simulink model "base_simulink"  (R2021b)
settings: Solver=FixedStepAuto  StartTime=0.0  StopTime=6  FixedStep=0.00005  RelTol=1e-3
undefined symbols (not defined in the file): sigbuilder_block, twist, X, Y, Z
libraries: sm_lib x128, nesl_utility x42, slpidlib x16, ros2lib x8
(part 1 of 6)
settings Model: Creator=sanpo  LastModifiedBy=matas
settings DebuggingCC: AlgebraicLoopMsg=none

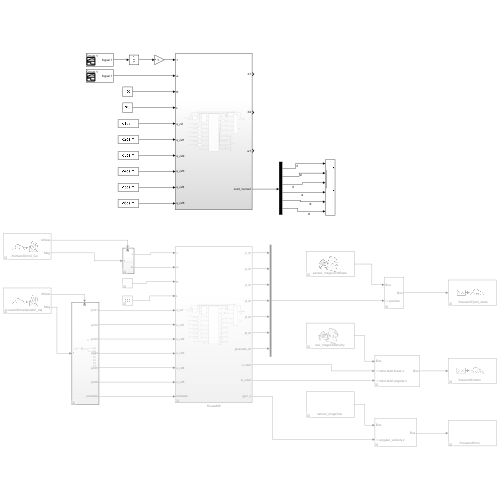
[thumbnail: Simulink's stored preview of the top-level diagram]
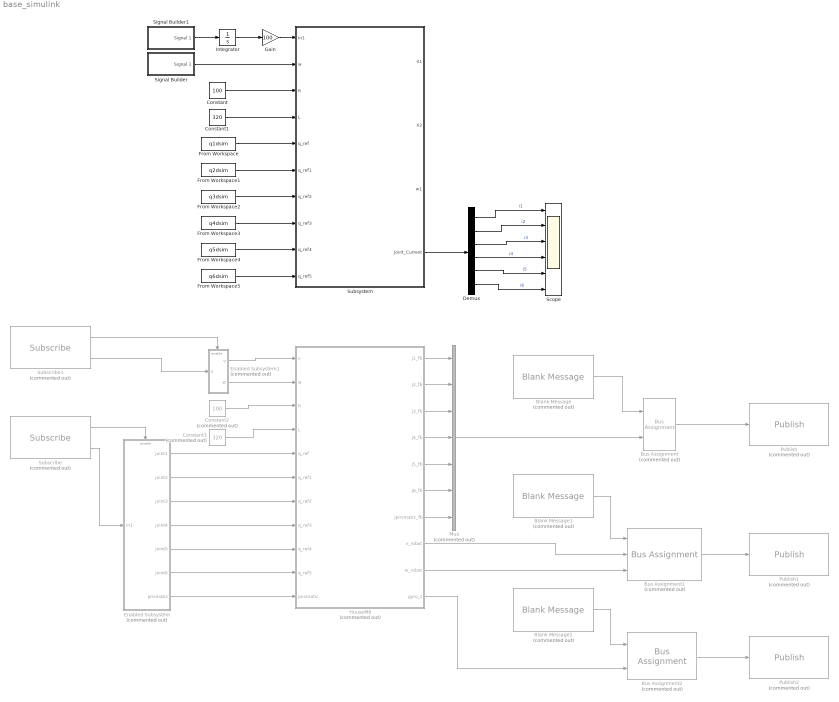
== system base_simulink ==
  Blank Message : ros2lib/Blank Message  Commented=on  messageClass=Message  entityType=sensor_msgs/JointState  messageType=sensor_msgs/JointState  SampleTime=0.01
      settings: SourceProductBaseCode=RR
  Blank Message1 : ros2lib/Blank Message  Commented=on  messageClass=Message  entityType=nav_msgs/Odometry  messageType=nav_msgs/Odometry  SampleTime=0.01
      settings: SourceProductBaseCode=RR
  Blank Message2 : ros2lib/Blank Message  Commented=on  messageClass=Message  entityType=sensor_msgs/Imu  messageType=geometry_msgs/Point  SampleTime=0.01
      settings: SourceProductBaseCode=RR
  Bus Assignment : BusAssignment  Commented=on  AssignedSignals=position
  Bus Assignment1 : BusAssignment  Commented=on  AssignedSignals=twist.twist.linear.x,twist.twist.angular.z
  Bus Assignment2 : BusAssignment  Commented=on  AssignedSignals=angular_velocity.z
  Constant : Constant  Value=100
  Constant1 : Constant  Value=320
  Constant2 : Constant  Commented=on  Value=100
  Constant3 : Constant  Commented=on  Value=320
  Demux : Demux  Outputs=6
  Enabled Subsystem : Subsystem  Commented=on
  Enabled Subsystem1 : Subsystem  Commented=on
  From Workspace : FromWorkspace  VariableName=q1dsim
  From Workspace1 : FromWorkspace  VariableName=q2dsim
  From Workspace2 : FromWorkspace  VariableName=q3dsim
  From Workspace3 : FromWorkspace  VariableName=q4dsim
  From Workspace4 : FromWorkspace  VariableName=q5dsim
  From Workspace5 : FromWorkspace  VariableName=q6dsim
  Gain : Gain  Gain=100
  HouseM8 : Subsystem  Commented=on
  Integrator : Integrator
  Mux : Mux  Commented=on  Inputs=7
  Publish : ros2lib/Publish  Commented=on  topicSource=Specify your own  topic=/housem8/joint_state  messageType=sensor_msgs/JointState  QOSHistory=Keep last  QOSDepth=1  QOSReliability=Reliable  QOSDurability=Volatile
      settings: SourceProductBaseCode=RR
  Publish1 : ros2lib/Publish  Commented=on  topicSource=Specify your own  topic=/housem8/odom  messageType=geometry_msgs/Point  QOSHistory=Keep last  QOSDepth=1  QOSReliability=Reliable  QOSDurability=Volatile
      settings: SourceProductBaseCode=RR
  Publish2 : ros2lib/Publish  Commented=on  topicSource=Specify your own  topic=/housem8/imu  messageType=geometry_msgs/Point  QOSHistory=Keep last  QOSDepth=1  QOSReliability=Reliable  QOSDurability=Volatile
      settings: SourceProductBaseCode=RR
  Scope : Scope  NumInputPorts=6
  Signal Builder : Subsystem  Tag=STV Subsys  LoadFcn=sigbuilder_block('load');  StartFcn=sigbuilder_block('start');  StopFcn=sigbuilder_block('stop');  ClipboardFcn=sigbuilder_block('clipboard');  mask(Sigbuilder block){tuvar=[0:10]}
      mask help: Simulink:masks:SigbuilderBlock_MD
      mask init:
      | if ~strcmp(get_param(bdroot(gcbh),'SimulationStatus'),'stopped') tuvar = sigbuilder_block('maskInit'); end
      settings: CopyFcn=sigbuilder_block('copy');  DeleteFcn=sigbuilder_block('delete');  ModelCloseFcn=sigbuilder_block('modelClose');  PreSaveFcn=sigbuilder_block('preSave');  PauseFcn=sigbuilder_block('pause');  ContinueFcn=sigbuilder_block('continue');  NameChangeFcn=sigbuilder_block('namechange');  OpenFcn=sigbuilder_block('open',[543 204.75 550.5 399.75 ]);  CloseFcn=sigbuilder_block('close');
      mask Display: plot(0, 0, 100, 100,[2, 2, 32, 32, 2], [68, 8, 8, 68, 68],[32, 2], [38, 38], [32, 19, 2],[53, 60, 44], [32, 17, 17, 2],[16, 16, 31, 31]);txt = getActiveGroup(gcbh);text(2, 100, txt,'verticalAlignment', 'top');
  Signal Builder1 : Subsystem  Tag=STV Subsys  LoadFcn=sigbuilder_block('load');  StartFcn=sigbuilder_block('start');  StopFcn=sigbuilder_block('stop');  ClipboardFcn=sigbuilder_block('clipboard');  mask(Sigbuilder block){tuvar=[0:10]}
      mask help: Simulink:masks:SigbuilderBlock_MD
      mask init:
      | if ~strcmp(get_param(bdroot(gcbh),'SimulationStatus'),'stopped') tuvar = sigbuilder_block('maskInit'); end
      settings: CopyFcn=sigbuilder_block('copy');  DeleteFcn=sigbuilder_block('delete');  ModelCloseFcn=sigbuilder_block('modelClose');  PreSaveFcn=sigbuilder_block('preSave');  PauseFcn=sigbuilder_block('pause');  ContinueFcn=sigbuilder_block('continue');  NameChangeFcn=sigbuilder_block('namechange');  OpenFcn=sigbuilder_block('open',[543 204.75 550.5 399.75 ]);  CloseFcn=sigbuilder_block('close');
      mask Display: plot(0, 0, 100, 100,[2, 2, 32, 32, 2], [68, 8, 8, 68, 68],[32, 2], [38, 38], [32, 19, 2],[53, 60, 44], [32, 17, 17, 2],[16, 16, 31, 31]);txt = getActiveGroup(gcbh);text(2, 100, txt,'verticalAlignment', 'top');
  Subscribe : ros2lib/Subscribe  Commented=on  topicSource=Specify your own  topic=/housem8/manipulator_traj  messageType=trajectory_msgs/MultiDOFJointTrajectory  sampleTime=0.01  QOSHistory=Keep last  QOSDepth=1  QOSReliability=Reliable  QOSDurability=Volatile
      settings: SourceProductBaseCode=RR
  Subscribe1 : ros2lib/Subscribe  Commented=on  topicSource=Specify your own  topic=/homem8/cmd_vel  messageType=geometry_msgs/Twist  sampleTime=0.01  QOSHistory=Keep last  QOSDepth=1  QOSReliability=Reliable  QOSDurability=Volatile
      settings: SourceProductBaseCode=RR
  Subsystem : Subsystem
  wires:
  Integrator/1 -> Gain/1
  Signal Builder1/1(Signal 1) -> Integrator/1
  Gain/1 -> Subsystem/1(In1)
  Signal Builder/1(Signal 1) -> Subsystem/2(w)
  Constant/1 -> Subsystem/3(R)
  Constant1/1 -> Subsystem/4(L)
  From Workspace/1 -> Subsystem/5(q_ref)
  From Workspace1/1 -> Subsystem/6(q_ref1)
  From Workspace2/1 -> Subsystem/7(q_ref2)
  From Workspace3/1 -> Subsystem/8(q_ref3)
  From Workspace4/1 -> Subsystem/9(q_ref4)
  From Workspace5/1 -> Subsystem/10(q_ref5)
  Subscribe/2 -> Enabled Subsystem/1(In1)
  Subscribe/1 -> Enabled Subsystem/Enable
  Constant3/1 -> HouseM8/4(L)
  Constant2/1 -> HouseM8/3(R)
  Enabled Subsystem/7(prismatic) -> HouseM8/11(prismatic)
  Enabled Subsystem/1(่่joint1) -> HouseM8/5(q_ref)
  Enabled Subsystem/2(joint2) -> HouseM8/6(q_ref1)
  Enabled Subsystem/3(joint3) -> HouseM8/7(q_ref2)
  Enabled Subsystem/4(joint4) -> HouseM8/8(q_ref3)
  Enabled Subsystem/5(joint5) -> HouseM8/9(q_ref4)
  Enabled Subsystem/6(joint6) -> HouseM8/10(q_ref5)
  Blank Message/1 -> Bus Assignment/1
  Bus Assignment/1 -> Publish/1
  Bus Assignment1/1 -> Publish1/1
  Blank Message1/1 -> Bus Assignment1/1
  Bus Assignment2/1 -> Publish2/1
  Blank Message2/1 -> Bus Assignment2/1
  HouseM8/10(gyro_z) -> Bus Assignment2/2
  HouseM8/1(j1_fb) -> Mux/1
  HouseM8/3(j3_fb) -> Mux/3
  HouseM8/2(j2_fb) -> Mux/2
  HouseM8/4(j4_fb) -> Mux/4
  HouseM8/5(j5_fb) -> Mux/5
  HouseM8/6(j6_fb) -> Mux/6
  HouseM8/7(jprismatic_fb) -> Mux/7
  Mux/1 -> Bus Assignment/2
  HouseM8/8(v_robot) -> Bus Assignment1/2
  HouseM8/9(w_robot) -> Bus Assignment1/3
  Subscribe1/1 -> Enabled Subsystem1/Enable
  Subscribe1/2 -> Enabled Subsystem1/1(In1)
  Enabled Subsystem1/1(v) -> HouseM8/1(v)
  Enabled Subsystem1/2(w) -> HouseM8/2(w)
  Subsystem/4(Joint_Current) -> Demux/1
  Demux/1 -> Scope/1  "i1"
  Demux/2 -> Scope/2  "i2"
  Demux/3 -> Scope/3  "i3"
  Demux/4 -> Scope/4  "i4"
  Demux/5 -> Scope/5  "i5"
  Demux/6 -> Scope/6  "i6"

== system base_simulink/Enabled Subsystem ==
  In1 : Inport
  Enable : EnablePort
  Bus Selector : BusSelector  DialogController=Simulink.DDGSource_BusSelector  OutputSignals=x,y
  ่่joint1 : Outport  VectorParamsAs1DForOutWhenUnconnected=off
  joint2 : Outport  Port=2  VectorParamsAs1DForOutWhenUnconnected=off
  joint3 : Outport  Port=3  VectorParamsAs1DForOutWhenUnconnected=off
  joint4 : Outport  Port=4  VectorParamsAs1DForOutWhenUnconnected=off
  joint5 : Outport  Port=5  VectorParamsAs1DForOutWhenUnconnected=off
  joint6 : Outport  Port=6  VectorParamsAs1DForOutWhenUnconnected=off
  prismatic : Outport  Port=7  VectorParamsAs1DForOutWhenUnconnected=off
  wires:
  In1/1 -> Bus Selector/1
  Bus Selector/1 -> ่่joint1/1  "<x>"
  Bus Selector/2 -> joint2/1  "<y>"

== system base_simulink/Enabled Subsystem1 ==
  In1 : Inport
  Enable : EnablePort
  Bus Selector : BusSelector  DialogController=Simulink.DDGSource_BusSelector  OutputSignals=x,y
  v : Outport  VectorParamsAs1DForOutWhenUnconnected=off
  w : Outport  Port=2  VectorParamsAs1DForOutWhenUnconnected=off
  wires:
  In1/1 -> Bus Selector/1
  Bus Selector/1 -> v/1  "<x>"
  Bus Selector/2 -> w/1  "<y>"

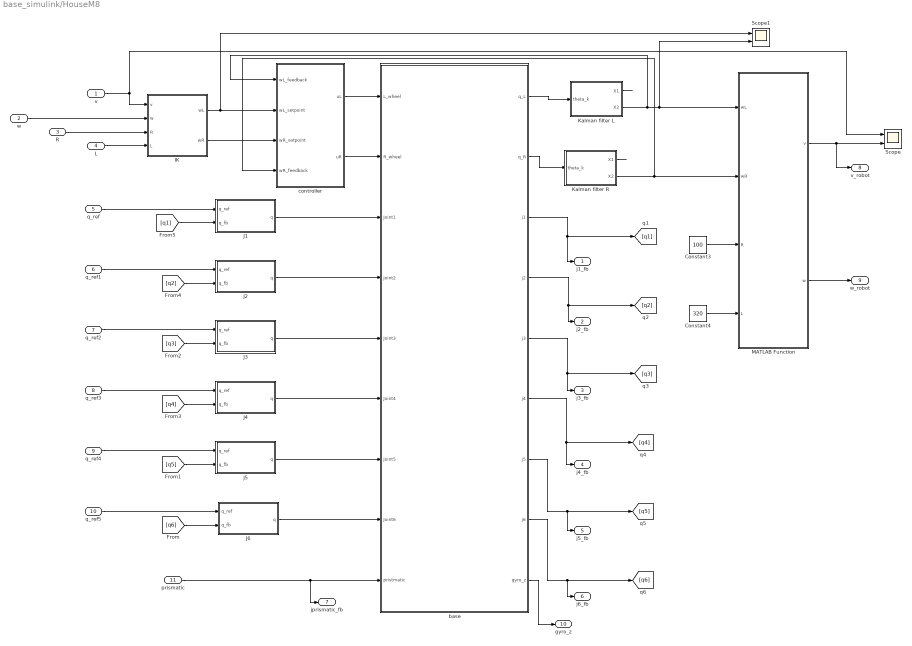
== system base_simulink/HouseM8 ==
  v : Inport
  w : Inport  Port=2
  R : Inport  Port=3
  L : Inport  Port=4
  q_ref : Inport  Port=5
  q_ref1 : Inport  Port=6
  q_ref2 : Inport  Port=7
  q_ref3 : Inport  Port=8
  q_ref4 : Inport  Port=9
  q_ref5 : Inport  Port=10
  prismatic : Inport  Port=11
  Constant3 : Constant  Value=100
  Constant4 : Constant  Value=320
  IK : MATLAB Function  TreatAsAtomicUnit=on
  J1 : Subsystem
  J2 : Subsystem
  J3 : Subsystem
  J4 : Subsystem
  J5 : Subsystem
  J6 : Subsystem
  Kalman filter L : Subsystem
  Kalman filter R : Subsystem
  MATLAB Function : MATLAB Function  TreatAsAtomicUnit=on
  Scope : Scope  NumInputPorts=2
  Scope1 : Scope  NumInputPorts=2
  base : Subsystem
  controller : Subsystem
  j1_fb : Outport
  j2_fb : Outport  Port=2
  j3_fb : Outport  Port=3
  j4_fb : Outport  Port=4
  j5_fb : Outport  Port=5
  j6_fb : Outport  Port=6
  jprismatic_fb : Outport  Port=7
  v_robot : Outport  Port=8
  w_robot : Outport  Port=9
  gyro_z : Outport  Port=10
  wires:
  base/4(j2) -> j2_fb/1, [q2]
  v/1 -> Scope/1, IK/1(v)
  IK/1(wL) -> Scope1/1, controller/2(wL_setpoint)
  Constant4/1 -> MATLAB Function/4(L)
  J6/1(q) -> base/8(Joint6)
  Kalman filter R/2(X2) -> controller/4(wR_feedback), MATLAB Function/2(wR)
  J1/1(q) -> base/3(Joint1)
  controller/2(uR) -> base/2(R_wheel)
  Kalman filter L/2(X2) -> Scope1/2, MATLAB Function/1(wL), controller/1(wL_feedback)
  base/8(j6) -> j6_fb/1, [q6]
  MATLAB Function/1(v) -> v_robot/1, Scope/2
  base/5(j3) -> j3_fb/1, [q3]
  q_ref2/1 -> J3/1(q_ref)
  base/2(q_R) -> Kalman filter R/1(theta_k)
  L/1 -> IK/4(L)
  J3/1(q) -> base/5(Joint3)
  Constant3/1 -> MATLAB Function/3(R)
  base/1(q_L) -> Kalman filter L/1(theta_k)
  q_ref/1 -> J1/1(q_ref)
  q_ref1/1 -> J2/1(q_ref)
  IK/2(wR) -> controller/3(wR_setpoint)
  Kalman filter L/1(X1) -> ?
  base/3(j1) -> j1_fb/1, [q1]
  prismatic/1 -> jprismatic_fb/1, base/9(pristmatic)
  [q1] -> J1/2(q_fb)
  q_ref5/1 -> J6/1(q_ref)
  base/6(j4) -> j4_fb/1, [q4]
  controller/1(uL) -> base/1(L_wheel)
  [q5] -> J5/2(q_fb)
  J4/1(q) -> base/6(Joint4)
  base/7(j5) -> j5_fb/1, [q5]
  [q2] -> J2/2(q_fb)
  [q3] -> J3/2(q_fb)
  J2/1(q) -> base/4(Joint2)
  Kalman filter R/1(X1) -> ?
  J5/1(q) -> base/7(Joint5)
  [q4] -> J4/2(q_fb)
  [q6] -> J6/2(q_fb)
  R/1 -> IK/3(R)
  w/1 -> IK/2(w)
  q_ref4/1 -> J5/1(q_ref)
  q_ref3/1 -> J4/1(q_ref)
  MATLAB Function/2(w) -> w_robot/1
  base/9(gyro_z) -> gyro_z/1

== system base_simulink/Signal Builder ==
  Demux : Demux  Tag=STV Demux  Outputs=1
      settings: DisplayOption=none
  FromWs : FromWorkspace  Tag=STV FromWs  VariableName=tuvar
      SigBuilderData=|
      | common.afterFinalStr = 'Extrapolate'
      | common.sampleTime = 0
      | dataSet.timeRange = [0 10]
      | dataSet.name = 'Group 1'
      | sbobj.Groups.Name = 'Group 1'
      | sbobj.Groups.Signals.Name = 'Signal 1'
      | sbobj.Groups.Signals.XData = [0 2 3 4 5 6 10]
      | sbobj.Groups.Signals.YData = [0 0 1 1 0 0 -1]
      | sbobj.Groups.TimeRange = [0 10]
  Signal 1 : Outport  Tag=STV Outport
  wires:
  Demux/1 -> Signal 1/1
  FromWs/1 -> Demux/1

== system base_simulink/Signal Builder1 ==
  Demux : Demux  Tag=STV Demux  Outputs=1
      settings: DisplayOption=none
  FromWs : FromWorkspace  Tag=STV FromWs  VariableName=tuvar
      SigBuilderData=|
      | common.afterFinalStr = 'Extrapolate'
      | common.sampleTime = 0
      | dataSet.timeRange = [0 10]
      | dataSet.name = 'Group 1'
      | sbobj.Groups.Name = 'Group 1'
      | sbobj.Groups.Signals.Name = 'Signal 1'
      | sbobj.Groups.Signals.XData = [0 0.5 6 10]
      | sbobj.Groups.Signals.YData = [5e-10 0.5 1 0]
  Signal 1 : Outport  Tag=STV Outport
  wires:
  FromWs/1 -> Demux/1
  Demux/1 -> Signal 1/1

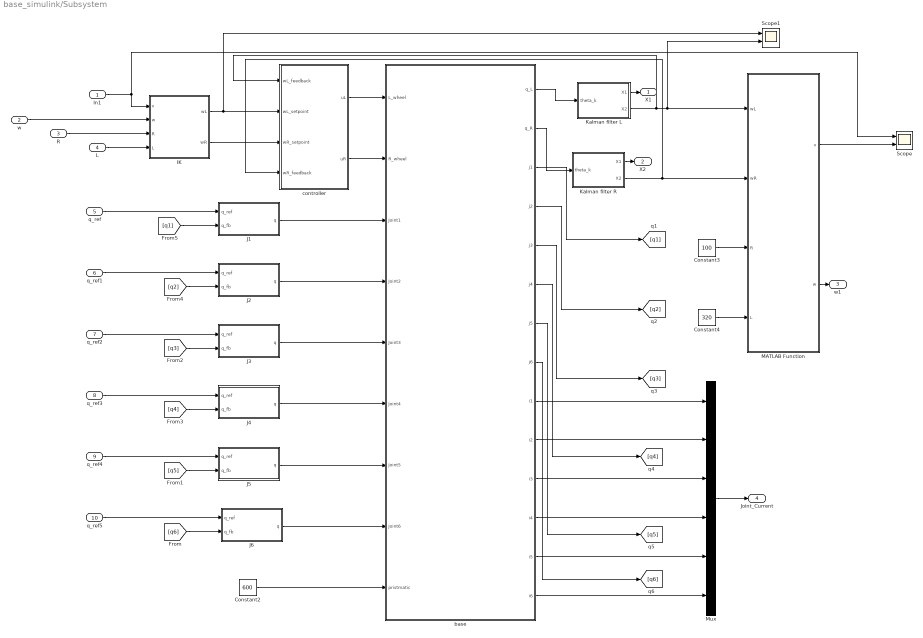
== system base_simulink/Subsystem ==
  In1 : Inport
  w : Inport  Port=2
  R : Inport  Port=3
  L : Inport  Port=4
  q_ref : Inport  Port=5
  q_ref1 : Inport  Port=6
  q_ref2 : Inport  Port=7
  q_ref3 : Inport  Port=8
  q_ref4 : Inport  Port=9
  q_ref5 : Inport  Port=10
  Constant2 : Constant  Value=600
  Constant3 : Constant  Value=100
  Constant4 : Constant  Value=320
  IK : MATLAB Function  TreatAsAtomicUnit=on
  J1 : Subsystem
  J2 : Subsystem
  J3 : Subsystem
  J4 : Subsystem
  J5 : Subsystem
  J6 : Subsystem
  Kalman filter L : Subsystem
  Kalman filter R : Subsystem
  MATLAB Function : MATLAB Function  TreatAsAtomicUnit=on
  Mux : Mux  Inputs=6
  Scope : Scope  NumInputPorts=2
  Scope1 : Scope  NumInputPorts=2
  base : Subsystem
  controller : Subsystem
  X1 : Outport
  X2 : Outport  Port=2
  w1 : Outport  Port=3
  Joint_Current : Outport  Port=4
  wires:
  base/4(j2) -> [q2]
  In1/1 -> Scope/1, IK/1(v)
  IK/1(wL) -> Scope1/1, controller/2(wL_setpoint)
  Constant4/1 -> MATLAB Function/4(L)
  J6/1(q) -> base/8(Joint6)
  Kalman filter R/2(X2) -> controller/4(wR_feedback), MATLAB Function/2(wR)
  J1/1(q) -> base/3(Joint1)
  controller/2(uR) -> base/2(R_wheel)
  Kalman filter L/2(X2) -> Scope1/2, MATLAB Function/1(wL), controller/1(wL_feedback)
  base/8(j6) -> [q6]
  MATLAB Function/1(v) -> Scope/2
  base/5(j3) -> [q3]
  q_ref2/1 -> J3/1(q_ref)
  base/2(q_R) -> Kalman filter R/1(theta_k)
  L/1 -> IK/4(L)
  J3/1(q) -> base/5(Joint3)
  Constant3/1 -> MATLAB Function/3(R)
  base/1(q_L) -> Kalman filter L/1(theta_k)
  q_ref/1 -> J1/1(q_ref)
  q_ref1/1 -> J2/1(q_ref)
  IK/2(wR) -> controller/3(wR_setpoint)
  Kalman filter L/1(X1) -> X1/1
  base/3(j1) -> [q1]
  Constant2/1 -> base/9(pristmatic)
  [q1] -> J1/2(q_fb)
  q_ref5/1 -> J6/1(q_ref)
  base/6(j4) -> [q4]
  controller/1(uL) -> base/1(L_wheel)
  [q5] -> J5/2(q_fb)
  J4/1(q) -> base/6(Joint4)
  base/7(j5) -> [q5]
  [q2] -> J2/2(q_fb)
  [q3] -> J3/2(q_fb)
  J2/1(q) -> base/4(Joint2)
  Kalman filter R/1(X1) -> X2/1
  J5/1(q) -> base/7(Joint5)
  [q4] -> J4/2(q_fb)
  [q6] -> J6/2(q_fb)
  R/1 -> IK/3(R)
  w/1 -> IK/2(w)
  q_ref4/1 -> J5/1(q_ref)
  q_ref3/1 -> J4/1(q_ref)
  MATLAB Function/2(w) -> w1/1
  base/9(i1) -> Mux/1
  base/10(i2) -> Mux/2
  base/11(i3) -> Mux/3
  base/12(i4) -> Mux/4
  base/13(i5) -> Mux/5
  base/14(i6) -> Mux/6
  Mux/1 -> Joint_Current/1

== system base_simulink/HouseM8/J1 ==
  q_ref : Inport
  q_fb : Inport  Port=2
  PID Controller : slpidlib/PID Controller  Controller=PID  Form=Parallel  TimeDomain=Discrete-time  UseExternalTs=off  SampleTime=0.001  IntegratorMethod=Forward Euler  FilterMethod=Forward Euler  ControllerParametersSource=internal  P=80  I=30  D=10  UseFilter=on  N=100  TunerSelectOption=Transfer Function Based (PID Tuner App)  InitialConditionSource=internal  InitialConditionForIntegrator=0  InitialConditionForFilter=0  DifferentiatorICPrevScaledInput=0  ExternalReset=none  TrackingMode=off  Kt=1  LimitOutput=off  SatLimitsSource=internal  UpperSaturationLimit=inf  LowerSaturationLimit=-inf  LinearizeAsGain=on  AntiWindupMode=none  Kb=1  POutMin=[]  POutMax=[]  IOutMin=[]  IOutMax=[]  DOutMin=[]  DOutMax=[]  NOutMin=[]  NOutMax=[]  SumOutMin=[]  SumOutMax=[]  SaturationOutMin=[]  SaturationOutMax=[]  PParamMin=[]  PParamMax=[]  IParamMin=[]  IParamMax=[]  DParamMin=[]  DParamMax=[]  NParamMin=[]  NParamMax=[]  KbParamMin=[]  KbParamMax=[]  KtParamMin=[]  KtParamMax=[]  KbOutMin=[]  KbOutMax=[]  KtOutMin=[]  KtOutMax=[]  IntegratorOutMin=[]  IntegratorOutMax=[]  FilterOutMin=[]  FilterOutMax=[]  SumI1OutMin=[]  SumI1OutMax=[]  SumI2OutMin=[]  SumI2OutMax=[]  SumI3OutMin=[]  SumI3OutMax=[]  SumI4OutMin=[]  SumI4OutMax=[]  SumDOutMin=[]  SumDOutMax=[]  DifferentiatorOutMin=[]  DifferentiatorOutMax=[]  FilterDiffOutCoefMin=[]  FilterDiffOutCoefMax=[]  ReciprocalOutMin=[]  ReciprocalOutMax=[]  SumDenOutMin=[]  SumDenOutMax=[]  SumNumOutMin=[]  SumNumOutMax=[]  DivideOutMin=[]  DivideOutMax=[]  UdiffTsProdOutMin=[]  UdiffTsProdOutMax=[]  NTsProdOutMin=[]  NTsProdOutMax=[]  UintegralTsProdOutMin=[]  UintegralTsProdOutMax=[]  UngainTsProdOutMin=[]  UngainTsProdOutMax=[]  IntegratorContinuousStateAttributes=''  IntegratorStateMustResolveToSignalObject=off  IntegratorRTWStateStorageClass=Auto  FilterContinuousStateAttributes=''  FilterStateMustResolveToSignalObject=off  FilterRTWStateStorageClass=Auto  ParallelPVariant=InternalParameters  IdealPVariant=Disabled  IVariant=InternalParameters  DVariant=InternalParameters  IntegratorVariant=Discrete  SatVariant=Disabled  AWVariant=Passthrough  PCopyVariant=Disabled  TRVariant=Disabled  FdbkBlocksVariant=Forward  IdealPFdbkVariant=Disabled  SatFdbkVariant=Disabled  DerivativeFilterVariant=ForwardEulerFilter  NVariant=InternalParameters  NCopyVariant=Disabled  FilterICVariant=InternalICsFilter  IntegratorICVariant=InternalICs  ExternalResetVariant=Disabled  TRSumVariant=Passthrough  SumFdbkVariant=Disabled  SumVariant=Sum_PID  TsampFilterVariant=InternalTs  TsampNgainVariant=Passthrough  TsampIntegralVariant=Passthrough  ExternalSaturationOutDataTypeStr=Inherit: Same as second input
  Sum : Sum  Inputs=|+-
  q : Outport
  wires:
  PID Controller/1 -> q/1
  Sum/1 -> PID Controller/1
  q_ref/1 -> Sum/1
  q_fb/1 -> Sum/2

== system base_simulink/HouseM8/J2 ==
  q_ref : Inport
  q_fb : Inport  Port=2
  PID Controller : slpidlib/PID Controller  Controller=PID  Form=Parallel  TimeDomain=Discrete-time  UseExternalTs=off  SampleTime=0.001  IntegratorMethod=Forward Euler  FilterMethod=Forward Euler  ControllerParametersSource=internal  P=90  I=30  D=12  UseFilter=on  N=100  TunerSelectOption=Transfer Function Based (PID Tuner App)  InitialConditionSource=internal  InitialConditionForIntegrator=0  InitialConditionForFilter=0  DifferentiatorICPrevScaledInput=0  ExternalReset=none  TrackingMode=off  Kt=1  LimitOutput=off  SatLimitsSource=internal  UpperSaturationLimit=inf  LowerSaturationLimit=-inf  LinearizeAsGain=on  AntiWindupMode=none  Kb=1  POutMin=[]  POutMax=[]  IOutMin=[]  IOutMax=[]  DOutMin=[]  DOutMax=[]  NOutMin=[]  NOutMax=[]  SumOutMin=[]  SumOutMax=[]  SaturationOutMin=[]  SaturationOutMax=[]  PParamMin=[]  PParamMax=[]  IParamMin=[]  IParamMax=[]  DParamMin=[]  DParamMax=[]  NParamMin=[]  NParamMax=[]  KbParamMin=[]  KbParamMax=[]  KtParamMin=[]  KtParamMax=[]  KbOutMin=[]  KbOutMax=[]  KtOutMin=[]  KtOutMax=[]  IntegratorOutMin=[]  IntegratorOutMax=[]  FilterOutMin=[]  FilterOutMax=[]  SumI1OutMin=[]  SumI1OutMax=[]  SumI2OutMin=[]  SumI2OutMax=[]  SumI3OutMin=[]  SumI3OutMax=[]  SumI4OutMin=[]  SumI4OutMax=[]  SumDOutMin=[]  SumDOutMax=[]  DifferentiatorOutMin=[]  DifferentiatorOutMax=[]  FilterDiffOutCoefMin=[]  FilterDiffOutCoefMax=[]  ReciprocalOutMin=[]  ReciprocalOutMax=[]  SumDenOutMin=[]  SumDenOutMax=[]  SumNumOutMin=[]  SumNumOutMax=[]  DivideOutMin=[]  DivideOutMax=[]  UdiffTsProdOutMin=[]  UdiffTsProdOutMax=[]  NTsProdOutMin=[]  NTsProdOutMax=[]  UintegralTsProdOutMin=[]  UintegralTsProdOutMax=[]  UngainTsProdOutMin=[]  UngainTsProdOutMax=[]  IntegratorContinuousStateAttributes=''  IntegratorStateMustResolveToSignalObject=off  IntegratorRTWStateStorageClass=Auto  FilterContinuousStateAttributes=''  FilterStateMustResolveToSignalObject=off  FilterRTWStateStorageClass=Auto  ParallelPVariant=InternalParameters  IdealPVariant=Disabled  IVariant=InternalParameters  DVariant=InternalParameters  IntegratorVariant=Discrete  SatVariant=Disabled  AWVariant=Passthrough  PCopyVariant=Disabled  TRVariant=Disabled  FdbkBlocksVariant=Forward  IdealPFdbkVariant=Disabled  SatFdbkVariant=Disabled  DerivativeFilterVariant=ForwardEulerFilter  NVariant=InternalParameters  NCopyVariant=Disabled  FilterICVariant=InternalICsFilter  IntegratorICVariant=InternalICs  ExternalResetVariant=Disabled  TRSumVariant=Passthrough  SumFdbkVariant=Disabled  SumVariant=Sum_PID  TsampFilterVariant=InternalTs  TsampNgainVariant=Passthrough  TsampIntegralVariant=Passthrough  ExternalSaturationOutDataTypeStr=Inherit: Same as second input
  Scope : Scope  NumInputPorts=2
  Sum : Sum  Inputs=|+-
  q : Outport
  wires:
  PID Controller/1 -> q/1
  Sum/1 -> PID Controller/1
  q_ref/1 -> Scope/1, Sum/1
  q_fb/1 -> Scope/2, Sum/2

== system base_simulink/HouseM8/J3 ==
  q_ref : Inport
  q_fb : Inport  Port=2
  PID Controller : slpidlib/PID Controller  Controller=PID  Form=Parallel  TimeDomain=Discrete-time  UseExternalTs=off  SampleTime=0.001  IntegratorMethod=Forward Euler  FilterMethod=Forward Euler  ControllerParametersSource=internal  P=80  I=25  D=12  UseFilter=on  N=100  TunerSelectOption=Transfer Function Based (PID Tuner App)  InitialConditionSource=internal  InitialConditionForIntegrator=0  InitialConditionForFilter=0  DifferentiatorICPrevScaledInput=0  ExternalReset=none  TrackingMode=off  Kt=1  LimitOutput=off  SatLimitsSource=internal  UpperSaturationLimit=inf  LowerSaturationLimit=-inf  LinearizeAsGain=on  AntiWindupMode=none  Kb=1  POutMin=[]  POutMax=[]  IOutMin=[]  IOutMax=[]  DOutMin=[]  DOutMax=[]  NOutMin=[]  NOutMax=[]  SumOutMin=[]  SumOutMax=[]  SaturationOutMin=[]  SaturationOutMax=[]  PParamMin=[]  PParamMax=[]  IParamMin=[]  IParamMax=[]  DParamMin=[]  DParamMax=[]  NParamMin=[]  NParamMax=[]  KbParamMin=[]  KbParamMax=[]  KtParamMin=[]  KtParamMax=[]  KbOutMin=[]  KbOutMax=[]  KtOutMin=[]  KtOutMax=[]  IntegratorOutMin=[]  IntegratorOutMax=[]  FilterOutMin=[]  FilterOutMax=[]  SumI1OutMin=[]  SumI1OutMax=[]  SumI2OutMin=[]  SumI2OutMax=[]  SumI3OutMin=[]  SumI3OutMax=[]  SumI4OutMin=[]  SumI4OutMax=[]  SumDOutMin=[]  SumDOutMax=[]  DifferentiatorOutMin=[]  DifferentiatorOutMax=[]  FilterDiffOutCoefMin=[]  FilterDiffOutCoefMax=[]  ReciprocalOutMin=[]  ReciprocalOutMax=[]  SumDenOutMin=[]  SumDenOutMax=[]  SumNumOutMin=[]  SumNumOutMax=[]  DivideOutMin=[]  DivideOutMax=[]  UdiffTsProdOutMin=[]  UdiffTsProdOutMax=[]  NTsProdOutMin=[]  NTsProdOutMax=[]  UintegralTsProdOutMin=[]  UintegralTsProdOutMax=[]  UngainTsProdOutMin=[]  UngainTsProdOutMax=[]  IntegratorContinuousStateAttributes=''  IntegratorStateMustResolveToSignalObject=off  IntegratorRTWStateStorageClass=Auto  FilterContinuousStateAttributes=''  FilterStateMustResolveToSignalObject=off  FilterRTWStateStorageClass=Auto  ParallelPVariant=InternalParameters  IdealPVariant=Disabled  IVariant=InternalParameters  DVariant=InternalParameters  IntegratorVariant=Discrete  SatVariant=Disabled  AWVariant=Passthrough  PCopyVariant=Disabled  TRVariant=Disabled  FdbkBlocksVariant=Forward  IdealPFdbkVariant=Disabled  SatFdbkVariant=Disabled  DerivativeFilterVariant=ForwardEulerFilter  NVariant=InternalParameters  NCopyVariant=Disabled  FilterICVariant=InternalICsFilter  IntegratorICVariant=InternalICs  ExternalResetVariant=Disabled  TRSumVariant=Passthrough  SumFdbkVariant=Disabled  SumVariant=Sum_PID  TsampFilterVariant=InternalTs  TsampNgainVariant=Passthrough  TsampIntegralVariant=Passthrough  ExternalSaturationOutDataTypeStr=Inherit: Same as second input
  Scope : Scope  NumInputPorts=2
  Sum : Sum  Inputs=|+-
  q : Outport
  wires:
  PID Controller/1 -> q/1
  Sum/1 -> PID Controller/1
  q_ref/1 -> Scope/1, Sum/1
  q_fb/1 -> Scope/2, Sum/2

== system base_simulink/HouseM8/J4 ==
  q_ref : Inport
  q_fb : Inport  Port=2
  PID Controller : slpidlib/PID Controller  Controller=PID  Form=Parallel  TimeDomain=Discrete-time  UseExternalTs=off  SampleTime=0.001  IntegratorMethod=Forward Euler  FilterMethod=Forward Euler  ControllerParametersSource=internal  P=80  I=20  D=8  UseFilter=on  N=100  TunerSelectOption=Transfer Function Based (PID Tuner App)  InitialConditionSource=internal  InitialConditionForIntegrator=0  InitialConditionForFilter=0  DifferentiatorICPrevScaledInput=0  ExternalReset=none  TrackingMode=off  Kt=1  LimitOutput=off  SatLimitsSource=internal  UpperSaturationLimit=inf  LowerSaturationLimit=-inf  LinearizeAsGain=on  AntiWindupMode=none  Kb=1  POutMin=[]  POutMax=[]  IOutMin=[]  IOutMax=[]  DOutMin=[]  DOutMax=[]  NOutMin=[]  NOutMax=[]  SumOutMin=[]  SumOutMax=[]  SaturationOutMin=[]  SaturationOutMax=[]  PParamMin=[]  PParamMax=[]  IParamMin=[]  IParamMax=[]  DParamMin=[]  DParamMax=[]  NParamMin=[]  NParamMax=[]  KbParamMin=[]  KbParamMax=[]  KtParamMin=[]  KtParamMax=[]  KbOutMin=[]  KbOutMax=[]  KtOutMin=[]  KtOutMax=[]  IntegratorOutMin=[]  IntegratorOutMax=[]  FilterOutMin=[]  FilterOutMax=[]  SumI1OutMin=[]  SumI1OutMax=[]  SumI2OutMin=[]  SumI2OutMax=[]  SumI3OutMin=[]  SumI3OutMax=[]  SumI4OutMin=[]  SumI4OutMax=[]  SumDOutMin=[]  SumDOutMax=[]  DifferentiatorOutMin=[]  DifferentiatorOutMax=[]  FilterDiffOutCoefMin=[]  FilterDiffOutCoefMax=[]  ReciprocalOutMin=[]  ReciprocalOutMax=[]  SumDenOutMin=[]  SumDenOutMax=[]  SumNumOutMin=[]  SumNumOutMax=[]  DivideOutMin=[]  DivideOutMax=[]  UdiffTsProdOutMin=[]  UdiffTsProdOutMax=[]  NTsProdOutMin=[]  NTsProdOutMax=[]  UintegralTsProdOutMin=[]  UintegralTsProdOutMax=[]  UngainTsProdOutMin=[]  UngainTsProdOutMax=[]  IntegratorContinuousStateAttributes=''  IntegratorStateMustResolveToSignalObject=off  IntegratorRTWStateStorageClass=Auto  FilterContinuousStateAttributes=''  FilterStateMustResolveToSignalObject=off  FilterRTWStateStorageClass=Auto  ParallelPVariant=InternalParameters  IdealPVariant=Disabled  IVariant=InternalParameters  DVariant=InternalParameters  IntegratorVariant=Discrete  SatVariant=Disabled  AWVariant=Passthrough  PCopyVariant=Disabled  TRVariant=Disabled  FdbkBlocksVariant=Forward  IdealPFdbkVariant=Disabled  SatFdbkVariant=Disabled  DerivativeFilterVariant=ForwardEulerFilter  NVariant=InternalParameters  NCopyVariant=Disabled  FilterICVariant=InternalICsFilter  IntegratorICVariant=InternalICs  ExternalResetVariant=Disabled  TRSumVariant=Passthrough  SumFdbkVariant=Disabled  SumVariant=Sum_PID  TsampFilterVariant=InternalTs  TsampNgainVariant=Passthrough  TsampIntegralVariant=Passthrough  ExternalSaturationOutDataTypeStr=Inherit: Same as second input
  Scope : Scope  NumInputPorts=2
  Sum : Sum  Inputs=|+-
  q : Outport
  wires:
  PID Controller/1 -> q/1
  Sum/1 -> PID Controller/1
  q_ref/1 -> Scope/1, Sum/1
  q_fb/1 -> Scope/2, Sum/2

== system base_simulink/HouseM8/J5 ==
  q_ref : Inport
  q_fb : Inport  Port=2
  PID Controller : slpidlib/PID Controller  Controller=PID  Form=Parallel  TimeDomain=Discrete-time  UseExternalTs=off  SampleTime=0.001  IntegratorMethod=Forward Euler  FilterMethod=Forward Euler  ControllerParametersSource=internal  P=85  I=25  D=10  UseFilter=on  N=100  TunerSelectOption=Transfer Function Based (PID Tuner App)  InitialConditionSource=internal  InitialConditionForIntegrator=0  InitialConditionForFilter=0  DifferentiatorICPrevScaledInput=0  ExternalReset=none  TrackingMode=off  Kt=1  LimitOutput=off  SatLimitsSource=internal  UpperSaturationLimit=inf  LowerSaturationLimit=-inf  LinearizeAsGain=on  AntiWindupMode=none  Kb=1  POutMin=[]  POutMax=[]  IOutMin=[]  IOutMax=[]  DOutMin=[]  DOutMax=[]  NOutMin=[]  NOutMax=[]  SumOutMin=[]  SumOutMax=[]  SaturationOutMin=[]  SaturationOutMax=[]  PParamMin=[]  PParamMax=[]  IParamMin=[]  IParamMax=[]  DParamMin=[]  DParamMax=[]  NParamMin=[]  NParamMax=[]  KbParamMin=[]  KbParamMax=[]  KtParamMin=[]  KtParamMax=[]  KbOutMin=[]  KbOutMax=[]  KtOutMin=[]  KtOutMax=[]  IntegratorOutMin=[]  IntegratorOutMax=[]  FilterOutMin=[]  FilterOutMax=[]  SumI1OutMin=[]  SumI1OutMax=[]  SumI2OutMin=[]  SumI2OutMax=[]  SumI3OutMin=[]  SumI3OutMax=[]  SumI4OutMin=[]  SumI4OutMax=[]  SumDOutMin=[]  SumDOutMax=[]  DifferentiatorOutMin=[]  DifferentiatorOutMax=[]  FilterDiffOutCoefMin=[]  FilterDiffOutCoefMax=[]  ReciprocalOutMin=[]  ReciprocalOutMax=[]  SumDenOutMin=[]  SumDenOutMax=[]  SumNumOutMin=[]  SumNumOutMax=[]  DivideOutMin=[]  DivideOutMax=[]  UdiffTsProdOutMin=[]  UdiffTsProdOutMax=[]  NTsProdOutMin=[]  NTsProdOutMax=[]  UintegralTsProdOutMin=[]  UintegralTsProdOutMax=[]  UngainTsProdOutMin=[]  UngainTsProdOutMax=[]  IntegratorContinuousStateAttributes=''  IntegratorStateMustResolveToSignalObject=off  IntegratorRTWStateStorageClass=Auto  FilterContinuousStateAttributes=''  FilterStateMustResolveToSignalObject=off  FilterRTWStateStorageClass=Auto  ParallelPVariant=InternalParameters  IdealPVariant=Disabled  IVariant=InternalParameters  DVariant=InternalParameters  IntegratorVariant=Discrete  SatVariant=Disabled  AWVariant=Passthrough  PCopyVariant=Disabled  TRVariant=Disabled  FdbkBlocksVariant=Forward  IdealPFdbkVariant=Disabled  SatFdbkVariant=Disabled  DerivativeFilterVariant=ForwardEulerFilter  NVariant=InternalParameters  NCopyVariant=Disabled  FilterICVariant=InternalICsFilter  IntegratorICVariant=InternalICs  ExternalResetVariant=Disabled  TRSumVariant=Passthrough  SumFdbkVariant=Disabled  SumVariant=Sum_PID  TsampFilterVariant=InternalTs  TsampNgainVariant=Passthrough  TsampIntegralVariant=Passthrough  ExternalSaturationOutDataTypeStr=Inherit: Same as second input
  Scope : Scope  NumInputPorts=2
  Sum : Sum  Inputs=|+-
  q : Outport
  wires:
  PID Controller/1 -> q/1
  Sum/1 -> PID Controller/1
  q_ref/1 -> Scope/1, Sum/1
  q_fb/1 -> Scope/2, Sum/2

== system base_simulink/HouseM8/J6 ==
  q_ref : Inport
  q_fb : Inport  Port=2
  PID Controller : slpidlib/PID Controller  Controller=PID  Form=Parallel  TimeDomain=Discrete-time  UseExternalTs=off  SampleTime=0.001  IntegratorMethod=Forward Euler  FilterMethod=Forward Euler  ControllerParametersSource=internal  P=65  I=32  D=10  UseFilter=on  N=100  TunerSelectOption=Transfer Function Based (PID Tuner App)  InitialConditionSource=internal  InitialConditionForIntegrator=0  InitialConditionForFilter=0  DifferentiatorICPrevScaledInput=0  ExternalReset=none  TrackingMode=off  Kt=1  LimitOutput=off  SatLimitsSource=internal  UpperSaturationLimit=inf  LowerSaturationLimit=-inf  LinearizeAsGain=on  AntiWindupMode=none  Kb=1  POutMin=[]  POutMax=[]  IOutMin=[]  IOutMax=[]  DOutMin=[]  DOutMax=[]  NOutMin=[]  NOutMax=[]  SumOutMin=[]  SumOutMax=[]  SaturationOutMin=[]  SaturationOutMax=[]  PParamMin=[]  PParamMax=[]  IParamMin=[]  IParamMax=[]  DParamMin=[]  DParamMax=[]  NParamMin=[]  NParamMax=[]  KbParamMin=[]  KbParamMax=[]  KtParamMin=[]  KtParamMax=[]  KbOutMin=[]  KbOutMax=[]  KtOutMin=[]  KtOutMax=[]  IntegratorOutMin=[]  IntegratorOutMax=[]  FilterOutMin=[]  FilterOutMax=[]  SumI1OutMin=[]  SumI1OutMax=[]  SumI2OutMin=[]  SumI2OutMax=[]  SumI3OutMin=[]  SumI3OutMax=[]  SumI4OutMin=[]  SumI4OutMax=[]  SumDOutMin=[]  SumDOutMax=[]  DifferentiatorOutMin=[]  DifferentiatorOutMax=[]  FilterDiffOutCoefMin=[]  FilterDiffOutCoefMax=[]  ReciprocalOutMin=[]  ReciprocalOutMax=[]  SumDenOutMin=[]  SumDenOutMax=[]  SumNumOutMin=[]  SumNumOutMax=[]  DivideOutMin=[]  DivideOutMax=[]  UdiffTsProdOutMin=[]  UdiffTsProdOutMax=[]  NTsProdOutMin=[]  NTsProdOutMax=[]  UintegralTsProdOutMin=[]  UintegralTsProdOutMax=[]  UngainTsProdOutMin=[]  UngainTsProdOutMax=[]  IntegratorContinuousStateAttributes=''  IntegratorStateMustResolveToSignalObject=off  IntegratorRTWStateStorageClass=Auto  FilterContinuousStateAttributes=''  FilterStateMustResolveToSignalObject=off  FilterRTWStateStorageClass=Auto  ParallelPVariant=InternalParameters  IdealPVariant=Disabled  IVariant=InternalParameters  DVariant=InternalParameters  IntegratorVariant=Discrete  SatVariant=Disabled  AWVariant=Passthrough  PCopyVariant=Disabled  TRVariant=Disabled  FdbkBlocksVariant=Forward  IdealPFdbkVariant=Disabled  SatFdbkVariant=Disabled  DerivativeFilterVariant=ForwardEulerFilter  NVariant=InternalParameters  NCopyVariant=Disabled  FilterICVariant=InternalICsFilter  IntegratorICVariant=InternalICs  ExternalResetVariant=Disabled  TRSumVariant=Passthrough  SumFdbkVariant=Disabled  SumVariant=Sum_PID  TsampFilterVariant=InternalTs  TsampNgainVariant=Passthrough  TsampIntegralVariant=Passthrough  ExternalSaturationOutDataTypeStr=Inherit: Same as second input
  Scope : Scope  NumInputPorts=2
  Sum : Sum  Inputs=|+-
  q : Outport
  wires:
  PID Controller/1 -> q/1
  Sum/1 -> PID Controller/1
  q_ref/1 -> Scope/1, Sum/1
  q_fb/1 -> Scope/2, Sum/2

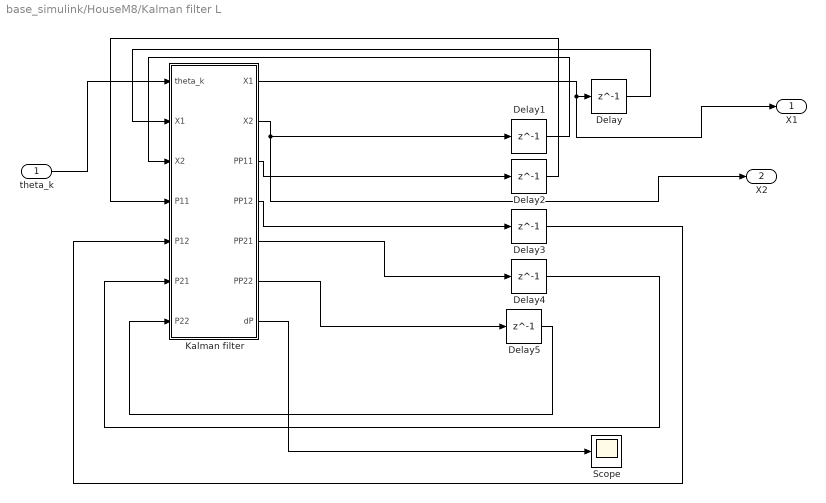
== system base_simulink/HouseM8/Kalman filter L ==
  theta_k : Inport
  Delay{,1..5} (6 alike) : Delay  DelayLength=1  SampleTime=0.0001
  Kalman filter : MATLAB Function  TreatAsAtomicUnit=on
  Scope : Scope
  X1 : Outport
  X2 : Outport  Port=2
  wires:
  Delay3/1 -> Kalman filter/5(P12)
  Kalman filter/3(PP11) -> Delay2/1
  Kalman filter/4(PP12) -> Delay3/1
  Delay2/1 -> Kalman filter/4(P11)
  Delay5/1 -> Kalman filter/7(P22)
  Delay/1 -> Kalman filter/2("X1 ")
  Kalman filter/1(X1) -> X1/1, Delay/1
  Kalman filter/5(PP21) -> Delay4/1
  Delay1/1 -> Kalman filter/3("X2 ")
  Delay4/1 -> Kalman filter/6(P21)
  theta_k/1 -> Kalman filter/1(theta_k)
  Kalman filter/2(X2) -> Delay1/1, X2/1
  Kalman filter/6(PP22) -> Delay5/1
  Kalman filter/7(dP) -> Scope/1

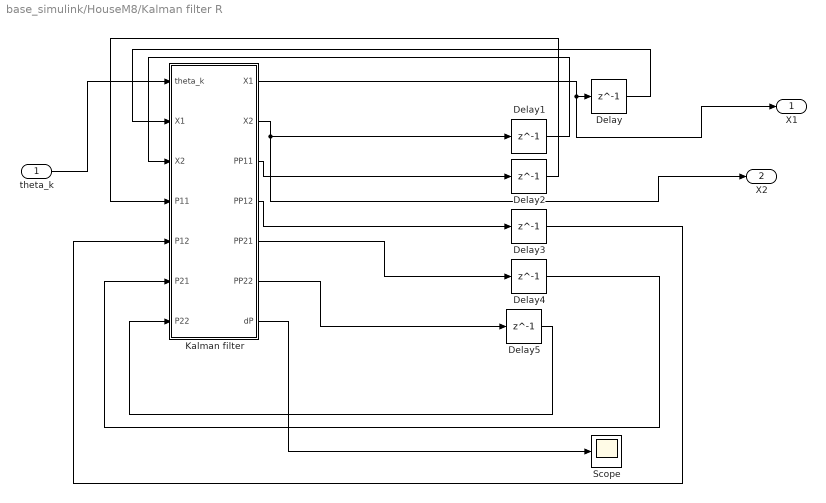
== system base_simulink/HouseM8/Kalman filter R ==
  theta_k : Inport
  Delay{,1..5} (6 alike) : Delay  DelayLength=1  SampleTime=0.0001
  Kalman filter : MATLAB Function  TreatAsAtomicUnit=on
  Scope : Scope
  X1 : Outport
  X2 : Outport  Port=2
  wires:
  Kalman filter/7(dP) -> Scope/1
  Kalman filter/6(PP22) -> Delay5/1
  Kalman filter/2(X2) -> X2/1, Delay1/1
  theta_k/1 -> Kalman filter/1(theta_k)
  Delay4/1 -> Kalman filter/6(P21)
  Delay1/1 -> Kalman filter/3("X2 ")
  Kalman filter/5(PP21) -> Delay4/1
  Kalman filter/1(X1) -> Delay/1, X1/1
  Delay/1 -> Kalman filter/2("X1 ")
  Delay5/1 -> Kalman filter/7(P22)
  Delay2/1 -> Kalman filter/4(P11)
  Kalman filter/4(PP12) -> Delay3/1
  Kalman filter/3(PP11) -> Delay2/1
  Delay3/1 -> Kalman filter/5(P12)

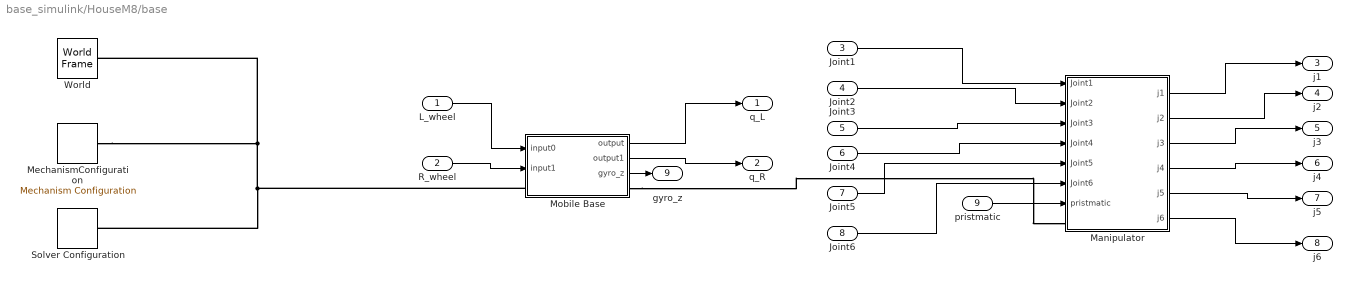
== system base_simulink/HouseM8/base ==
  L_wheel : Inport
  R_wheel : Inport  Port=2
  Joint1 : Inport  Port=3
  Joint2 : Inport  Port=4
  Joint3 : Inport  Port=5
  Joint4 : Inport  Port=6
  Joint5 : Inport  Port=7
  Joint6 : Inport  Port=8
  pristmatic : Inport  Port=9
  Manipulator : Subsystem
  MechanismConfiguration : sm_lib/Utilities/Mechanism Configuration  UniformGravity=Constant  GravityVector=[0 0 -9.80665]  GravityUnits=m/s^2  LinearizationDelta=0.001  JointModeTransitionNonlinearIterations=2
  Mobile Base : Subsystem
  Solver Configuration : nesl_utility/Solver Configuration  PhysicalDomain=network_engine_domain  SubClassName=solver  LeftPortType=input  RightPortType=generic  Tones=[]  Harmonics=[]  SimulateNoise=off  Profile=off  UseLocalSampling=off  EnableSwitchedLinearOptims=on  FrequencyDomain=off  UseCCode=off  RelTol=0.001  AbsTol=1e-06  MinStep=1e-09  ToWorkspace=off  RevertToSquareIcSolve=off  NumHomotopyIterations=100  PhasorMode=off  PhasorModeNumHarmonics=1  DoDC=off  ResidualTolerance=1e-09  UseLocalSolver=off  LocalSolverChoice=NE_BACKWARD_EULER_ADVANCER  LocalSolverSampleTime=0.001  DoFixedCost=off  MaxNonlinIter=3  MaxModeIter=2  ComputeImpulses=off  ImpulseIterations=2  LinearAlgebra=auto  EquationFormulation=NE_TIME_EF  DelaysMemoryBudget=1024  AutomaticFiltering=on  FilteringTimeConstant=0.001  PartitionStorageMethod=AS_NEEDED  PartitionMemoryBudget=1024  PartitionMethod=ROBUST
      settings: SourceProductBaseCode=PW,SS
  World : sm_lib/Frames and Transforms/World Frame
  q_L : Outport
  q_R : Outport  Port=2
  j1 : Outport  Port=3
  j2 : Outport  Port=4
  j3 : Outport  Port=5
  j4 : Outport  Port=6
  j5 : Outport  Port=7
  j6 : Outport  Port=8
  gyro_z : Outport  Port=9
  wires:
  L_wheel/1 -> Mobile Base/1(input0)
  R_wheel/1 -> Mobile Base/2(input1)
  Mobile Base/1(output) -> q_L/1
  Mobile Base/2(output1) -> q_R/1
  Joint1/1 -> Manipulator/1(Joint1)
  Joint2/1 -> Manipulator/2(Joint2)
  Joint3/1 -> Manipulator/3(Joint3)
  Joint4/1 -> Manipulator/4(Joint4)
  Joint5/1 -> Manipulator/5(Joint5)
  Joint6/1 -> Manipulator/6(Joint6)
  pristmatic/1 -> Manipulator/7(pristmatic)
  Manipulator/1(j1) -> j1/1
  Manipulator/2(j2) -> j2/1
  Manipulator/3(j3) -> j3/1
  Manipulator/4(j4) -> j4/1
  Manipulator/5(j5) -> j5/1
  Manipulator/6(j6) -> j6/1
  Mobile Base/3(gyro_z) -> gyro_z/1
  connections:
  Mobile Base/LConn1 -- Solver Configuration/RConn1 -- MechanismConfiguration/RConn1 -- World/RConn1
  Mobile Base/RConn1 -- Manipulator/LConn1

== system base_simulink/HouseM8/controller ==
  wL_feedback : Inport
  wL_setpoint : Inport  Port=2
  wR_setpoint : Inport  Port=3
  wR_feedback : Inport  Port=4
  PID Controller : slpidlib/PID Controller  Controller=PID  Form=Parallel  TimeDomain=Discrete-time  UseExternalTs=off  SampleTime=0.001  IntegratorMethod=Forward Euler  FilterMethod=Forward Euler  ControllerParametersSource=internal  P=1.5  I=0.6  D=1  UseFilter=on  N=100  TunerSelectOption=Transfer Function Based (PID Tuner App)  InitialConditionSource=internal  InitialConditionForIntegrator=0  InitialConditionForFilter=0  DifferentiatorICPrevScaledInput=0  ExternalReset=none  TrackingMode=off  Kt=1  LimitOutput=off  SatLimitsSource=internal  UpperSaturationLimit=inf  LowerSaturationLimit=-inf  LinearizeAsGain=on  AntiWindupMode=none  Kb=1  POutMin=[]  POutMax=[]  IOutMin=[]  IOutMax=[]  DOutMin=[]  DOutMax=[]  NOutMin=[]  NOutMax=[]  SumOutMin=[]  SumOutMax=[]  SaturationOutMin=[]  SaturationOutMax=[]  PParamMin=[]  PParamMax=[]  IParamMin=[]  IParamMax=[]  DParamMin=[]  DParamMax=[]  NParamMin=[]  NParamMax=[]  KbParamMin=[]  KbParamMax=[]  KtParamMin=[]  KtParamMax=[]  KbOutMin=[]  KbOutMax=[]  KtOutMin=[]  KtOutMax=[]  IntegratorOutMin=[]  IntegratorOutMax=[]  FilterOutMin=[]  FilterOutMax=[]  SumI1OutMin=[]  SumI1OutMax=[]  SumI2OutMin=[]  SumI2OutMax=[]  SumI3OutMin=[]  SumI3OutMax=[]  SumI4OutMin=[]  SumI4OutMax=[]  SumDOutMin=[]  SumDOutMax=[]  DifferentiatorOutMin=[]  DifferentiatorOutMax=[]  FilterDiffOutCoefMin=[]  FilterDiffOutCoefMax=[]  ReciprocalOutMin=[]  ReciprocalOutMax=[]  SumDenOutMin=[]  SumDenOutMax=[]  SumNumOutMin=[]  SumNumOutMax=[]  DivideOutMin=[]  DivideOutMax=[]  UdiffTsProdOutMin=[]  UdiffTsProdOutMax=[]  NTsProdOutMin=[]  NTsProdOutMax=[]  UintegralTsProdOutMin=[]  UintegralTsProdOutMax=[]  UngainTsProdOutMin=[]  UngainTsProdOutMax=[]  IntegratorContinuousStateAttributes=''  IntegratorStateMustResolveToSignalObject=off  IntegratorRTWStateStorageClass=Auto  FilterContinuousStateAttributes=''  FilterStateMustResolveToSignalObject=off  FilterRTWStateStorageClass=Auto  ParallelPVariant=InternalParameters  IdealPVariant=Disabled  IVariant=InternalParameters  DVariant=InternalParameters  IntegratorVariant=Discrete  SatVariant=Disabled  AWVariant=Passthrough  PCopyVariant=Disabled  TRVariant=Disabled  FdbkBlocksVariant=Forward  IdealPFdbkVariant=Disabled  SatFdbkVariant=Disabled  DerivativeFilterVariant=ForwardEulerFilter  NVariant=InternalParameters  NCopyVariant=Disabled  FilterICVariant=InternalICsFilter  IntegratorICVariant=InternalICs  ExternalResetVariant=Disabled  TRSumVariant=Passthrough  SumFdbkVariant=Disabled  SumVariant=Sum_PID  TsampFilterVariant=InternalTs  TsampNgainVariant=Passthrough  TsampIntegralVariant=Passthrough  ExternalSaturationOutDataTypeStr=Inherit: Same as second input
  PID Controller1 : slpidlib/PID Controller  Controller=PID  Form=Parallel  TimeDomain=Discrete-time  UseExternalTs=off  SampleTime=0.001  IntegratorMethod=Forward Euler  FilterMethod=Forward Euler  ControllerParametersSource=internal  P=1.5  I=0.6  D=1  UseFilter=on  N=100  TunerSelectOption=Transfer Function Based (PID Tuner App)  InitialConditionSource=internal  InitialConditionForIntegrator=0  InitialConditionForFilter=0  DifferentiatorICPrevScaledInput=0  ExternalReset=none  TrackingMode=off  Kt=1  LimitOutput=off  SatLimitsSource=internal  UpperSaturationLimit=inf  LowerSaturationLimit=-inf  LinearizeAsGain=on  AntiWindupMode=none  Kb=1  POutMin=[]  POutMax=[]  IOutMin=[]  IOutMax=[]  DOutMin=[]  DOutMax=[]  NOutMin=[]  NOutMax=[]  SumOutMin=[]  SumOutMax=[]  SaturationOutMin=[]  SaturationOutMax=[]  PParamMin=[]  PParamMax=[]  IParamMin=[]  IParamMax=[]  DParamMin=[]  DParamMax=[]  NParamMin=[]  NParamMax=[]  KbParamMin=[]  KbParamMax=[]  KtParamMin=[]  KtParamMax=[]  KbOutMin=[]  KbOutMax=[]  KtOutMin=[]  KtOutMax=[]  IntegratorOutMin=[]  IntegratorOutMax=[]  FilterOutMin=[]  FilterOutMax=[]  SumI1OutMin=[]  SumI1OutMax=[]  SumI2OutMin=[]  SumI2OutMax=[]  SumI3OutMin=[]  SumI3OutMax=[]  SumI4OutMin=[]  SumI4OutMax=[]  SumDOutMin=[]  SumDOutMax=[]  DifferentiatorOutMin=[]  DifferentiatorOutMax=[]  FilterDiffOutCoefMin=[]  FilterDiffOutCoefMax=[]  ReciprocalOutMin=[]  ReciprocalOutMax=[]  SumDenOutMin=[]  SumDenOutMax=[]  SumNumOutMin=[]  SumNumOutMax=[]  DivideOutMin=[]  DivideOutMax=[]  UdiffTsProdOutMin=[]  UdiffTsProdOutMax=[]  NTsProdOutMin=[]  NTsProdOutMax=[]  UintegralTsProdOutMin=[]  UintegralTsProdOutMax=[]  UngainTsProdOutMin=[]  UngainTsProdOutMax=[]  IntegratorContinuousStateAttributes=''  IntegratorStateMustResolveToSignalObject=off  IntegratorRTWStateStorageClass=Auto  FilterContinuousStateAttributes=''  FilterStateMustResolveToSignalObject=off  FilterRTWStateStorageClass=Auto  ParallelPVariant=InternalParameters  IdealPVariant=Disabled  IVariant=InternalParameters  DVariant=InternalParameters  IntegratorVariant=Discrete  SatVariant=Disabled  AWVariant=Passthrough  PCopyVariant=Disabled  TRVariant=Disabled  FdbkBlocksVariant=Forward  IdealPFdbkVariant=Disabled  SatFdbkVariant=Disabled  DerivativeFilterVariant=ForwardEulerFilter  NVariant=InternalParameters  NCopyVariant=Disabled  FilterICVariant=InternalICsFilter  IntegratorICVariant=InternalICs  ExternalResetVariant=Disabled  TRSumVariant=Passthrough  SumFdbkVariant=Disabled  SumVariant=Sum_PID  TsampFilterVariant=InternalTs  TsampNgainVariant=Passthrough  TsampIntegralVariant=Passthrough  ExternalSaturationOutDataTypeStr=Inherit: Same as second input
  Sum : Sum  Inputs=|+-
  Sum1 : Sum  Inputs=|+-
  uL : Outport
  uR : Outport  Port=2
  wires:
  PID Controller/1 -> uL/1
  Sum/1 -> PID Controller/1
  wL_setpoint/1 -> Sum/1
  wR_setpoint/1 -> Sum1/1
  Sum1/1 -> PID Controller1/1
  wR_feedback/1 -> Sum1/2
  PID Controller1/1 -> uR/1
  wL_feedback/1 -> Sum/2

== system base_simulink/Subsystem/J1 ==
  q_ref : Inport
  q_fb : Inport  Port=2
  PID Controller : slpidlib/PID Controller  Controller=PID  Form=Parallel  TimeDomain=Continuous-time  UseExternalTs=off  SampleTime=-1  IntegratorMethod=Forward Euler  FilterMethod=Forward Euler  ControllerParametersSource=internal  P=80  I=30  D=10  UseFilter=on  N=100  TunerSelectOption=Transfer Function Based (PID Tuner App)  InitialConditionSource=internal  InitialConditionForIntegrator=0  InitialConditionForFilter=0  DifferentiatorICPrevScaledInput=0  ExternalReset=none  TrackingMode=off  Kt=1  LimitOutput=off  SatLimitsSource=internal  UpperSaturationLimit=inf  LowerSaturationLimit=-inf  LinearizeAsGain=on  AntiWindupMode=none  Kb=1  POutMin=[]  POutMax=[]  IOutMin=[]  IOutMax=[]  DOutMin=[]  DOutMax=[]  NOutMin=[]  NOutMax=[]  SumOutMin=[]  SumOutMax=[]  SaturationOutMin=[]  SaturationOutMax=[]  PParamMin=[]  PParamMax=[]  IParamMin=[]  IParamMax=[]  DParamMin=[]  DParamMax=[]  NParamMin=[]  NParamMax=[]  KbParamMin=[]  KbParamMax=[]  KtParamMin=[]  KtParamMax=[]  KbOutMin=[]  KbOutMax=[]  KtOutMin=[]  KtOutMax=[]  IntegratorOutMin=[]  IntegratorOutMax=[]  FilterOutMin=[]  FilterOutMax=[]  SumI1OutMin=[]  SumI1OutMax=[]  SumI2OutMin=[]  SumI2OutMax=[]  SumI3OutMin=[]  SumI3OutMax=[]  SumI4OutMin=[]  SumI4OutMax=[]  SumDOutMin=[]  SumDOutMax=[]  DifferentiatorOutMin=[]  DifferentiatorOutMax=[]  FilterDiffOutCoefMin=[]  FilterDiffOutCoefMax=[]  ReciprocalOutMin=[]  ReciprocalOutMax=[]  SumDenOutMin=[]  SumDenOutMax=[]  SumNumOutMin=[]  SumNumOutMax=[]  DivideOutMin=[]  DivideOutMax=[]  UdiffTsProdOutMin=[]  UdiffTsProdOutMax=[]  NTsProdOutMin=[]  NTsProdOutMax=[]  UintegralTsProdOutMin=[]  UintegralTsProdOutMax=[]  UngainTsProdOutMin=[]  UngainTsProdOutMax=[]  IntegratorContinuousStateAttributes=''  IntegratorStateMustResolveToSignalObject=off  IntegratorRTWStateStorageClass=Auto  FilterContinuousStateAttributes=''  FilterStateMustResolveToSignalObject=off  FilterRTWStateStorageClass=Auto  ParallelPVariant=InternalParameters  IdealPVariant=Disabled  IVariant=InternalParameters  DVariant=InternalParameters  IntegratorVariant=Continuous  SatVariant=Disabled  AWVariant=Passthrough  PCopyVariant=Disabled  TRVariant=Disabled  FdbkBlocksVariant=Forward  IdealPFdbkVariant=Disabled  SatFdbkVariant=Disabled  DerivativeFilterVariant=ContFilter  NVariant=InternalParameters  NCopyVariant=Disabled  FilterICVariant=InternalICsFilter  IntegratorICVariant=InternalICs  ExternalResetVariant=Disabled  TRSumVariant=Passthrough  SumFdbkVariant=Disabled  SumVariant=Sum_PID  TsampFilterVariant=InternalTs  TsampNgainVariant=Passthrough  TsampIntegralVariant=Passthrough  ExternalSaturationOutDataTypeStr=Inherit: Same as second input
  Scope : Scope  NumInputPorts=2
  Sum : Sum  Inputs=|+-
  q : Outport
  wires:
  PID Controller/1 -> q/1
  Sum/1 -> PID Controller/1
  q_ref/1 -> Scope/1, Sum/1
  q_fb/1 -> Scope/2, Sum/2

== system base_simulink/Subsystem/J2 ==
  q_ref : Inport
  q_fb : Inport  Port=2
  PID Controller : slpidlib/PID Controller  Controller=PID  Form=Parallel  TimeDomain=Continuous-time  UseExternalTs=off  SampleTime=-1  IntegratorMethod=Forward Euler  FilterMethod=Forward Euler  ControllerParametersSource=internal  P=90  I=30  D=12  UseFilter=on  N=100  TunerSelectOption=Transfer Function Based (PID Tuner App)  InitialConditionSource=internal  InitialConditionForIntegrator=0  InitialConditionForFilter=0  DifferentiatorICPrevScaledInput=0  ExternalReset=none  TrackingMode=off  Kt=1  LimitOutput=off  SatLimitsSource=internal  UpperSaturationLimit=inf  LowerSaturationLimit=-inf  LinearizeAsGain=on  AntiWindupMode=none  Kb=1  POutMin=[]  POutMax=[]  IOutMin=[]  IOutMax=[]  DOutMin=[]  DOutMax=[]  NOutMin=[]  NOutMax=[]  SumOutMin=[]  SumOutMax=[]  SaturationOutMin=[]  SaturationOutMax=[]  PParamMin=[]  PParamMax=[]  IParamMin=[]  IParamMax=[]  DParamMin=[]  DParamMax=[]  NParamMin=[]  NParamMax=[]  KbParamMin=[]  KbParamMax=[]  KtParamMin=[]  KtParamMax=[]  KbOutMin=[]  KbOutMax=[]  KtOutMin=[]  KtOutMax=[]  IntegratorOutMin=[]  IntegratorOutMax=[]  FilterOutMin=[]  FilterOutMax=[]  SumI1OutMin=[]  SumI1OutMax=[]  SumI2OutMin=[]  SumI2OutMax=[]  SumI3OutMin=[]  SumI3OutMax=[]  SumI4OutMin=[]  SumI4OutMax=[]  SumDOutMin=[]  SumDOutMax=[]  DifferentiatorOutMin=[]  DifferentiatorOutMax=[]  FilterDiffOutCoefMin=[]  FilterDiffOutCoefMax=[]  ReciprocalOutMin=[]  ReciprocalOutMax=[]  SumDenOutMin=[]  SumDenOutMax=[]  SumNumOutMin=[]  SumNumOutMax=[]  DivideOutMin=[]  DivideOutMax=[]  UdiffTsProdOutMin=[]  UdiffTsProdOutMax=[]  NTsProdOutMin=[]  NTsProdOutMax=[]  UintegralTsProdOutMin=[]  UintegralTsProdOutMax=[]  UngainTsProdOutMin=[]  UngainTsProdOutMax=[]  IntegratorContinuousStateAttributes=''  IntegratorStateMustResolveToSignalObject=off  IntegratorRTWStateStorageClass=Auto  FilterContinuousStateAttributes=''  FilterStateMustResolveToSignalObject=off  FilterRTWStateStorageClass=Auto  ParallelPVariant=InternalParameters  IdealPVariant=Disabled  IVariant=InternalParameters  DVariant=InternalParameters  IntegratorVariant=Continuous  SatVariant=Disabled  AWVariant=Passthrough  PCopyVariant=Disabled  TRVariant=Disabled  FdbkBlocksVariant=Forward  IdealPFdbkVariant=Disabled  SatFdbkVariant=Disabled  DerivativeFilterVariant=ContFilter  NVariant=InternalParameters  NCopyVariant=Disabled  FilterICVariant=InternalICsFilter  IntegratorICVariant=InternalICs  ExternalResetVariant=Disabled  TRSumVariant=Passthrough  SumFdbkVariant=Disabled  SumVariant=Sum_PID  TsampFilterVariant=InternalTs  TsampNgainVariant=Passthrough  TsampIntegralVariant=Passthrough  ExternalSaturationOutDataTypeStr=Inherit: Same as second input
  Scope : Scope  NumInputPorts=2
  Sum : Sum  Inputs=|+-
  q : Outport
  wires:
  PID Controller/1 -> q/1
  Sum/1 -> PID Controller/1
  q_ref/1 -> Scope/1, Sum/1
  q_fb/1 -> Scope/2, Sum/2
